simulink model "ControlledRectifiers"  (R2021a)
settings: Solver=VariableStepAuto  StartTime=0.0  StopTime=.1  FixedStep=.00001  MaxStep=.00001  RelTol=1e-3
libraries: spsVoltageMeasurementLib x27, spsThyristorLib x23, spsACVoltageSourceLib x11, spsCurrentMeasurementLib x10, spsSeriesRLCBranchLib x10, spspowerguiLib x2, spsDiodeLib x1
settings Model: Creator=User  LastModifiedBy=User

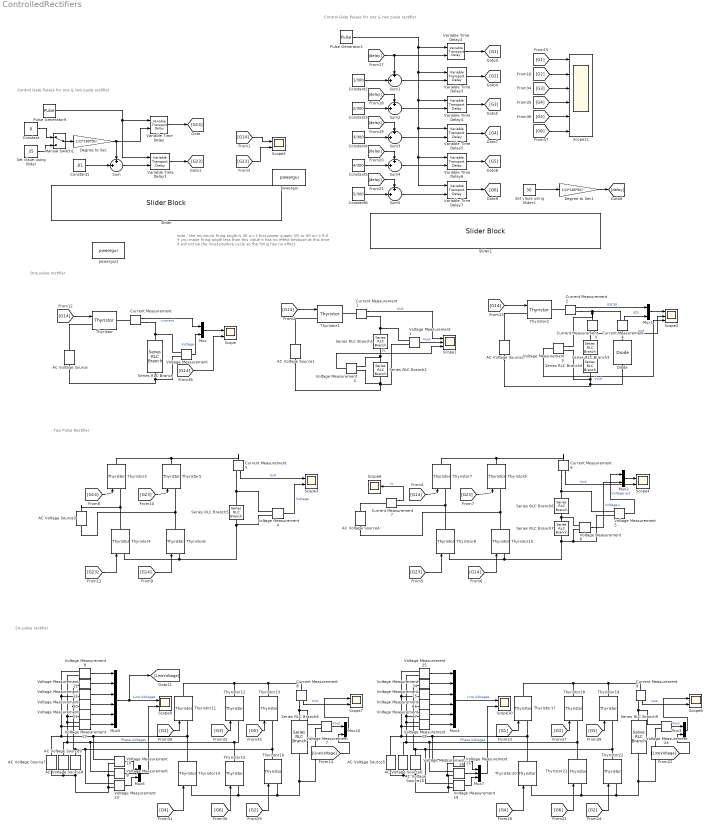
== system ControlledRectifiers ==
  note: Two Pulse Rectifier
  note: One pulse rectifier
  note: note :
      | the minimum firing angle is 30 w.r.t first power supply (R) or 60 w.r.t R-S if you make firing angle less than this value
      | it has no effect because at this time it will not be the most positive cycle so the firing has no effect
  note: Control Gate Pulses for one & two pusle rectifier
  note: Six pulse rectifier
  note: Control Gate Pulses for one & two pusle rectifier
  AC Voltage Source{,1..5,7} (7 alike) : spsACVoltageSourceLib/AC Voltage Source  Amplitude=220  Phase=0  Frequency=50  SampleTime=0  Measurements=None  BusType=swing  Pref=10e3  Qref=0  Qmin=-inf  Qmax=+inf
  AC Voltage Source10 : spsACVoltageSourceLib/AC Voltage Source  Amplitude=220  Phase=120  Frequency=50  SampleTime=0  Measurements=None  BusType=swing  Pref=10e3  Qref=0  Qmin=-inf  Qmax=+inf
  AC Voltage Source6 : spsACVoltageSourceLib/AC Voltage Source  Amplitude=220  Phase=-120  Frequency=50  SampleTime=0  Measurements=None  BusType=swing  Pref=10e3  Qref=0  Qmin=-inf  Qmax=+inf
  AC Voltage Source8 : spsACVoltageSourceLib/AC Voltage Source  Amplitude=220  Phase=-120  Frequency=50  SampleTime=0  Measurements=None  BusType=swing  Pref=10e3  Qref=0  Qmin=-inf  Qmax=+inf
  AC Voltage Source9 : spsACVoltageSourceLib/AC Voltage Source  Amplitude=220  Phase=120  Frequency=50  SampleTime=0  Measurements=None  BusType=swing  Pref=10e3  Qref=0  Qmin=-inf  Qmax=+inf
  Constant : Constant  Value=0
  Constant1 : Constant  Value=.01
  Constant2 : Constant  Value=1/300
  Constant3 : Constant  Value=2/300
  Constant4 : Constant  Value=3/300
  Constant5 : Constant  Value=4/300
  Constant6 : Constant  Value=5/300
  Current Measurement{,1..9} (10 alike) : spsCurrentMeasurementLib/Current Measurement  PhasorSimulation=off  OutputType=Complex  PSBequivalent=0
  Degree to Sec : Gain  Gain=1/(2*180*50)
  Degree to Sec1 : Gain  Gain=1/(2*180*50)
  Diode : spsDiodeLib/Diode  Ron=0.001  Lon=0  Vf=0.8  IC=0  UseSnubber=0  Rs=500  Cs=250e-9  Measurements=off
  Manual Switch1 : ManualSwitch
  Mux{,1..3,10} (5 alike) : Mux  Inputs=2
  Mux4 : Mux  Inputs=6
  Mux5 : Mux  Inputs=6
  Mux6 : Mux  Inputs=3
  Mux7 : Mux  Inputs=3
  Pulse Generator1 : DiscretePulseGenerator  PulseType=Time based  Period=.02  PulseWidth=5
  Pulse Generator9 : DiscretePulseGenerator  PulseType=Time based  Period=.02  PulseWidth=5
  Scope{,3..5,7..10} (8 alike) : Scope  NumInputPorts=2
  Scope1 : Scope  NumInputPorts=3
  Scope11 : Scope  NumInputPorts=6
  Scope2 : Scope  NumInputPorts=3
  Scope6 : Scope
  Series RLC Branch{,1,3,5,8..9} (6 alike) : spsSeriesRLCBranchLib/Series RLC Branch  LConnTagsString=__new0  RConnTagsString=__new0  BranchType=R  Resistance=10  Inductance=1e-3  SetiL0=off  InitialCurrent=0  Capacitance=1e-6  Setx0=off  InitialVoltage=0  Measurements=None
  Series RLC Branch2 : spsSeriesRLCBranchLib/Series RLC Branch  LConnTagsString=__new0  RConnTagsString=__new0  BranchType=L  Resistance=10  Inductance=100e-3  SetiL0=off  InitialCurrent=0  Capacitance=1e-6  Setx0=off  InitialVoltage=0  Measurements=None
  Series RLC Branch4 : spsSeriesRLCBranchLib/Series RLC Branch  LConnTagsString=__new0  RConnTagsString=__new0  BranchType=L  Resistance=10  Inductance=300e-3  SetiL0=off  InitialCurrent=0  Capacitance=1e-6  Setx0=off  InitialVoltage=0  Measurements=None
  Series RLC Branch6 : spsSeriesRLCBranchLib/Series RLC Branch  LConnTagsString=__new0  RConnTagsString=__new0  BranchType=R  Resistance=10  Inductance=100e-3  SetiL0=off  InitialCurrent=0  Capacitance=1e-6  Setx0=off  InitialVoltage=0  Measurements=None
  Series RLC Branch7 : spsSeriesRLCBranchLib/Series RLC Branch  LConnTagsString=__new0  RConnTagsString=__new0  BranchType=L  Resistance=10  Inductance=3  SetiL0=off  InitialCurrent=0  Capacitance=1e-6  Setx0=off  InitialVoltage=0  Measurements=None
  Set vlaue using Slider : Constant  Value=35
  Set vlaue using Slider1 : Constant  Value=30
  Slider : SliderBlock  ScaleMin=5  ScaleMax=180  TickInterval=5
  Slider1 : SliderBlock  ScaleMin=30  ScaleMax=180  TickInterval=5
  Sum{,1..5} (6 alike) : Sum  Inputs=+|+||
  Thyristor{,1..22} (23 alike) : spsThyristorLib/Thyristor  Ron=0.001  Lon=0  Vf=0.8  IC=0  Rs=500  Cs=250e-9  Measurements=off
  Variable Time Delay{,1..7} (8 alike) : VariableTransportDelay  MaximumDelay=10
  Voltage Measurement{,1..26} (27 alike) : spsVoltageMeasurementLib/Voltage Measurement  PhasorSimulation=off  OutputType=Complex  PSBequivalent=0
  powergui : spspowerguiLib/powergui  Priority=1  SimulationMode=Continuous  SampleTime=50e-6  frequency=60  Iterations=50  frequencyindice=50  Pbase=100e6  ErrMax=1e-4  UnitsV=kV  UnitsW=MW  buscounter=0  FunctionMessages=off  echomessages=off  EnableUseOfTLC=off  CurrentSourceSwitches=off  DisableSnubberDevices=off  DisableRonSwitches=off  DisableVfSwitches=off  DisplayEquations=off  AutomaticDiscreteSolvers=off  SolverType=Tustin/Backward Euler (TBE)  Interpol=off  ExternalGateDelay=off  methode=off  Ts=100  x0status=blocks  SPID=on  SwTol=0  HookPort=off  NonlinearTolerance=1e-4  nMaxIteration=100  ContinueOnMaxIteration=off  RestoreLinks=warning  ResistiveCurrentMeasurement=off  Frange=[0:2:500]  Ylog=off  Xlog=on  ShowGrid=off  save=off  variable=ZData  structure=0  ZoomFFT=off  StartTime=0.0  cycles=1  DisplayStyle=1  fundamental=60  FreqAxis=off  MaxFrequency=1000  frequencyindicesteady=1  RmsSteady=1  display=off
  powergui1 : spspowerguiLib/powergui  Priority=1  SimulationMode=Continuous  SampleTime=50e-6  frequency=60  Iterations=50  frequencyindice=50  Pbase=100e6  ErrMax=1e-4  UnitsV=kV  UnitsW=MW  buscounter=0  FunctionMessages=off  echomessages=off  EnableUseOfTLC=off  CurrentSourceSwitches=off  DisableSnubberDevices=off  DisableRonSwitches=off  DisableVfSwitches=off  DisplayEquations=off  AutomaticDiscreteSolvers=off  SolverType=Tustin/Backward Euler (TBE)  Interpol=off  ExternalGateDelay=off  methode=off  Ts=100  x0status=blocks  SPID=on  SwTol=0  HookPort=off  NonlinearTolerance=1e-4  nMaxIteration=100  ContinueOnMaxIteration=off  RestoreLinks=warning  ResistiveCurrentMeasurement=off  Frange=[0:2:500]  Ylog=off  Xlog=on  ShowGrid=off  save=off  variable=ZData  structure=0  ZoomFFT=off  StartTime=0.0  cycles=1  DisplayStyle=1  fundamental=60  FreqAxis=off  MaxFrequency=1000  frequencyindicesteady=1  RmsSteady=1  display=off
  wires:
  Mux/1 -> Scope/1
  Current Measurement/1 -> Mux/1  "currrent"
  Voltage Measurement/1 -> Mux/2  "Voltage"
  [G14] -> Thyristor/1
  [G14] -> Thyristor1/1
  Voltage Measurement1/1 -> Scope1/2  "Vout"
  Current Measurement1/1 -> Scope1/1  "Iout"
  Voltage Measurement2/1 -> Scope1/3  "VL"
  Current Measurement2/1 -> Mux1/1  "I(SCR)"
  [G14] -> Thyristor2/1
  Mux1/1 -> Scope2/1
  Current Measurement4/1 -> Mux1/2  "I(D)"
  Current Measurement3/1 -> Scope2/2  "Iout"
  Voltage Measurement3/1 -> Scope2/3  "Vout"
  [G14] -> Scope/2
  [G14] -> Thyristor3/1
  [G14] -> Thyristor6/1
  [G23] -> Thyristor5/1
  [G23] -> Thyristor4/1
  Current Measurement5/1 -> Scope3/1  "Iout"
  Voltage Measurement4/1 -> Scope3/2  "Voltage"
  Voltage Measurement5/1 -> Mux2/1  "Voltage out"
  Current Measurement6/1 -> Scope4/2  "Iout"
  [G23] -> Thyristor8/1
  [G23] -> Thyristor9/1
  [G14] -> Thyristor10/1
  [G14] -> Thyristor7/1
  Mux2/1 -> Scope4/1
  Voltage Measurement6/1 -> Mux2/2  "Voltage L"
  Pulse Generator9/1 -> Variable Time Delay1/1, Variable Time Delay/1
  Set vlaue using Slider/1 -> Manual Switch1/2
  Degree to Sec/1 -> Variable Time Delay/2, Sum/1
  Sum/1 -> Variable Time Delay1/2
  Constant1/1 -> Sum/2
  Variable Time Delay/1 -> [G14]
  Variable Time Delay1/1 -> [G23]
  [G14] -> Scope5/1
  [G23] -> Scope5/2
  Current Measurement7/1 -> Scope6/1  "Is"
  Mux10/1 -> Scope7/1
  [LineVoltage] -> Mux10/2
  Mux5/1 -> [LineVoltage], Scope9/1  "Line Voltages"
  Mux6/1 -> Scope9/2  "Phase Voltages"
  Voltage Measurement10/1 -> Mux6/1
  Voltage Measurement11/1 -> Mux5/2
  Voltage Measurement7/1 -> Mux10/1  "Vout"
  Current Measurement8/1 -> Scope7/2  "Iout"
  Voltage Measurement9/1 -> Mux6/2
  Voltage Measurement8/1 -> Mux5/1
  Voltage Measurement23/1 -> Mux6/3
  Voltage Measurement21/1 -> Mux5/5
  Voltage Measurement12/1 -> Mux5/3
  Voltage Measurement20/1 -> Mux5/4
  Voltage Measurement22/1 -> Mux5/6
  [G2] -> Scope11/2
  [G1] -> Scope11/1
  Variable Time Delay3/1 -> [G2]
  Variable Time Delay2/1 -> [G1]
  Constant2/1 -> Sum1/2
  Sum1/1 -> Variable Time Delay3/2
  Pulse Generator1/1 -> Variable Time Delay2/1, Variable Time Delay4/1, Variable Time Delay5/1, Variable Time Delay6/1, Variable Time Delay7/1, Variable Time Delay3/1
  Sum2/1 -> Variable Time Delay4/2
  Constant3/1 -> Sum2/2
  Variable Time Delay4/1 -> [G3]
  Degree to Sec1/1 -> [delay]
  [delay] -> Sum1/1, Variable Time Delay2/2
  [delay] -> Sum2/1
  [delay] -> Sum3/1
  Variable Time Delay5/1 -> [G4]
  Constant4/1 -> Sum3/2
  Sum3/1 -> Variable Time Delay5/2
  Sum4/1 -> Variable Time Delay6/2
  Constant5/1 -> Sum4/2
  Variable Time Delay6/1 -> [G5]
  [delay] -> Sum4/1
  [delay] -> Sum5/1
  Variable Time Delay7/1 -> [G6]
  Constant6/1 -> Sum5/2
  Sum5/1 -> Variable Time Delay7/2
  [G1] -> Thyristor11/1
  [G2] -> Thyristor16/1
  [G6] -> Thyristor15/1
  [G4] -> Thyristor14/1
  [G3] -> Thyristor12/1
  [G5] -> Thyristor13/1
  [G3] -> Scope11/3
  [G4] -> Scope11/4
  [G5] -> Scope11/5
  [G6] -> Scope11/6
  Constant/1 -> Manual Switch1/1
  [G5] -> Thyristor19/1
  [G3] -> Thyristor18/1
  [G4] -> Thyristor20/1
  [G6] -> Thyristor21/1
  [G2] -> Thyristor22/1
  [G1] -> Thyristor17/1
  Voltage Measurement18/1 -> Mux4/6
  Voltage Measurement16/1 -> Mux4/4
  Voltage Measurement15/1 -> Mux4/3
  Voltage Measurement17/1 -> Mux4/5
  Voltage Measurement19/1 -> Mux7/3
  Voltage Measurement25/1 -> Mux4/1
  Voltage Measurement26/1 -> Mux7/2
  Current Measurement9/1 -> Scope8/2  "Iout"
  Voltage Measurement24/1 -> Mux3/1  "Vout"
  Voltage Measurement14/1 -> Mux4/2
  Voltage Measurement13/1 -> Mux7/1
  Mux7/1 -> Scope10/2  "Phase Voltages"
  Mux4/1 -> Scope10/1  "Line Voltages"
  [LineVoltage] -> Mux3/2
  Mux3/1 -> Scope8/1
  Set vlaue using Slider1/1 -> Degree to Sec1/1
  Manual Switch1/1 -> Degree to Sec/1
  connections:
  Series RLC Branch/LConn1 -- Voltage Measurement/LConn1 -- Current Measurement/RConn1
  Series RLC Branch/RConn1 -- AC Voltage Source/LConn1 -- Voltage Measurement/LConn2
  Current Measurement/LConn1 -- Thyristor/RConn1
  Thyristor/LConn1 -- AC Voltage Source/RConn1
  Series RLC Branch1/LConn1 -- Current Measurement1/RConn1 -- Voltage Measurement1/LConn1
  AC Voltage Source1/LConn1 -- Voltage Measurement1/LConn2 -- Voltage Measurement2/LConn2 -- Series RLC Branch2/RConn1
  Current Measurement1/LConn1 -- Thyristor1/RConn1
  Thyristor1/LConn1 -- AC Voltage Source1/RConn1
  Series RLC Branch2/LConn1 -- Series RLC Branch1/RConn1 -- Voltage Measurement2/LConn1
  AC Voltage Source2/LConn1 -- Diode/LConn1 -- Voltage Measurement3/LConn2 -- Series RLC Branch4/RConn1
  Series RLC Branch4/LConn1 -- Series RLC Branch3/RConn1
  Thyristor2/LConn1 -- AC Voltage Source2/RConn1
  Current Measurement2/LConn1 -- Thyristor2/RConn1
  Current Measurement3/RConn1 -- Series RLC Branch3/LConn1
  Current Measurement2/RConn1 -- Current Measurement4/RConn1 -- Voltage Measurement3/LConn1 -- Current Measurement3/LConn1
  Diode/RConn1 -- Current Measurement4/LConn1
  Thyristor4/RConn1 -- AC Voltage Source3/RConn1 -- Thyristor3/LConn1
  Thyristor6/RConn1 -- AC Voltage Source3/LConn1 -- Thyristor5/LConn1
  Series RLC Branch5/LConn1 -- Current Measurement5/RConn1 -- Voltage Measurement4/LConn1
  Thyristor4/LConn1 -- Voltage Measurement4/LConn2 -- Series RLC Branch5/RConn1 -- Thyristor6/LConn1
  Current Measurement5/LConn1 -- Thyristor5/RConn1 -- Thyristor3/RConn1
  Thyristor7/LConn1 -- Current Measurement7/RConn1 -- Thyristor8/RConn1
  AC Voltage Source4/LConn1 -- Thyristor10/RConn1 -- Thyristor9/LConn1
  Current Measurement6/RConn1 -- Voltage Measurement5/LConn1 -- Series RLC Branch6/LConn1
  Voltage Measurement5/LConn2 -- Series RLC Branch7/RConn1 -- Thyristor10/LConn1 -- Thyristor8/LConn1 -- Voltage Measurement6/LConn2
  Current Measurement6/LConn1 -- Thyristor7/RConn1 -- Thyristor9/RConn1
  Series RLC Branch6/RConn1 -- Series RLC Branch7/LConn1 -- Voltage Measurement6/LConn1
  Current Measurement7/LConn1 -- AC Voltage Source4/RConn1
  Current Measurement8/LConn1 -- Thyristor11/RConn1 -- Thyristor12/RConn1 -- Thyristor13/RConn1
  AC Voltage Source7/LConn1 -- AC Voltage Source8/LConn1 -- AC Voltage Source9/LConn1 -- Voltage Measurement10/LConn2 -- Voltage Measurement9/LConn2 -- Voltage Measurement23/LConn2
  Voltage Measurement8/LConn1 -- AC Voltage Source7/RConn1 -- Thyristor14/RConn1 -- Thyristor11/LConn1 -- Voltage Measurement10/LConn1 -- Voltage Measurement22/LConn2 -- Voltage Measurement20/LConn1 -- Voltage Measurement12/LConn2
  Voltage Measurement9/LConn1 -- Thyristor12/LConn1 -- Thyristor15/RConn1 -- AC Voltage Source8/RConn1 -- Voltage Measurement22/LConn1 -- Voltage Measurement8/LConn2 -- Voltage Measurement11/LConn1 -- Voltage Measurement21/LConn2
  Voltage Measurement11/LConn2 -- Voltage Measurement12/LConn1 -- AC Voltage Source9/RConn1 -- Thyristor13/LConn1 -- Thyristor16/RConn1 -- Voltage Measurement23/LConn1 -- Voltage Measurement21/LConn1 -- Voltage Measurement20/LConn2
  Series RLC Branch8/RConn1 -- Thyristor14/LConn1 -- Thyristor15/LConn1 -- Thyristor16/LConn1 -- Voltage Measurement7/LConn2
  Current Measurement8/RConn1 -- Series RLC Branch8/LConn1 -- Voltage Measurement7/LConn1
  Current Measurement9/LConn1 -- Thyristor19/RConn1 -- Thyristor18/RConn1 -- Thyristor17/RConn1
  AC Voltage Source5/LConn1 -- Voltage Measurement19/LConn2 -- Voltage Measurement26/LConn2 -- Voltage Measurement13/LConn2 -- AC Voltage Source10/LConn1 -- AC Voltage Source6/LConn1
  Voltage Measurement25/LConn1 -- Voltage Measurement15/LConn2 -- Voltage Measurement16/LConn1 -- Voltage Measurement18/LConn2 -- Voltage Measurement13/LConn1 -- Thyristor20/RConn1 -- Thyristor17/LConn1 -- AC Voltage Source5/RConn1
  Voltage Measurement26/LConn1 -- Voltage Measurement17/LConn2 -- Voltage Measurement14/LConn1 -- Voltage Measurement25/LConn2 -- Voltage Measurement18/LConn1 -- AC Voltage Source6/RConn1 -- Thyristor18/LConn1 -- Thyristor21/RConn1
  Voltage Measurement14/LConn2 -- Voltage Measurement16/LConn2 -- Voltage Measurement17/LConn1 -- Voltage Measurement19/LConn1 -- Thyristor19/LConn1 -- Thyristor22/RConn1 -- AC Voltage Source10/RConn1 -- Voltage Measurement15/LConn1
  Series RLC Branch9/RConn1 -- Voltage Measurement24/LConn2 -- Thyristor20/LConn1 -- Thyristor21/LConn1 -- Thyristor22/LConn1
  Current Measurement9/RConn1 -- Voltage Measurement24/LConn1 -- Series RLC Branch9/LConn1
